simulink model "IEEE13NF_bal"  (Simulink 8.5)
settings: Solver=ode4  StartTime=0.0  StopTime=8  FixedStep=Ts  RelTol=1e-3
PreLoadFcn:
  | Ts=0.01;
PostLoadFcn:
  | Ts=0.01;
InitFcn:
  | Ts=0.01;
StartFcn:
  | Ts=0.01;
libraries: dspindex x5, opal_lib x2, rtlab x2, rtlab_phasor x1
settings Model: Creator=ZhiqiZhao  LastModifiedBy=Jaimie.Swartz
settings DebuggingCC: SolverPrmCheckMsg=warning  FcnCallInpInsideContextMsg=EnableAllAsWarning

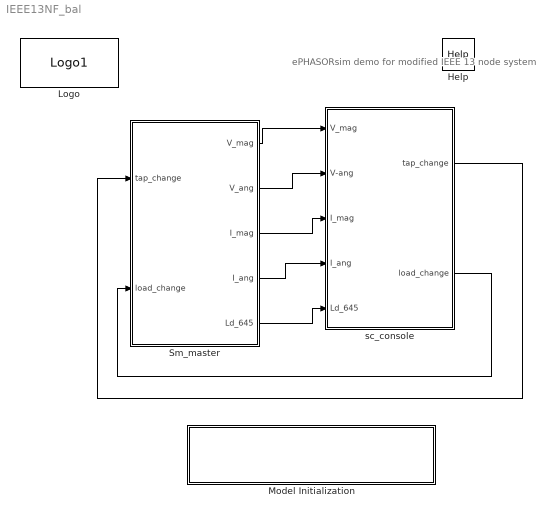
== system IEEE13NF_bal ==
  note: ePHASORsim demo for
      | modified IEEE 13 node system
  Help : opal_lib/Help  docfile=../help/ePH_IEEE13.html
  Logo : opal_lib/Logo1  vide=[]
  Model Initialization : Subsystem  mask(Model Functions){InitFcnX=Ts=0.01;, prel=on, posl=on, inif=on, strf=on}
      mask prompts: InitFcnX "Initialisation"; prel "Preload Function"; posl "PostLoad Function"; inif "InitFcn"; strf "StartFcn"
      mask init:
      | currentBlock = gcb;
      | root = bdroot(currentBlock);
      | 
      | if ~strcmp(get_param(root,'BlockDiagramType'),'library')
      |     if prel==1
      |         set_param(root, 'PreLoadFcn', InitFcnX);
      |     else
      |         set_param(root, 'PreLoadFcn', '');
      |     end
      |     if inif==1
      |         set_param(root, 'InitFcn', InitFcnX);
      |     else
      |         set_param(root, 'InitFcn', '');
      |     end
      |     if strf==1
      |         set_param(root, 'StartFcn', InitFcnX);
      |     else
      |         set_param(root, 'StartFcn', '');
      |     end
      |     if posl==1
      |         set_param(root, 'PostLoadFcn', InitFcnX);
      |     else
      |         set_param(root, 'PostLoadFcn', '');
      |     end
      | end
      | 
      | pos = get_param(currentBlock, 'Position');
      | width = pos(3) - pos(1); height = pos(4) - pos(2);
      | txt = [ upper(root) '\n' '- InitFcn. . . . . '  get_param(root, 'InitFcn') ];
      settings: CopyFcn=set_param(gcb,'LinkStatus','none')
      mask Display: text(5, height*0.5, txt, 'horizontalAlignment', 'left', 'verticalAlignment', 'middle') ;
  Sm_master : Subsystem
  sc_console : Subsystem
  wires:
  sc_console/1(tap_change) -> Sm_master/1(tap_change)
  sc_console/2(load_change) -> Sm_master/2(load_change)
  Sm_master/1(V_mag) -> sc_console/1(V_mag)
  Sm_master/2(V_ang) -> sc_console/2(V-ang)
  Sm_master/3(I_mag) -> sc_console/3(I_mag)
  Sm_master/4(I_ang) -> sc_console/4(I_ang)
  Sm_master/5(Ld_645) -> sc_console/5(Ld_645)

== system IEEE13NF_bal/Model Initialization ==

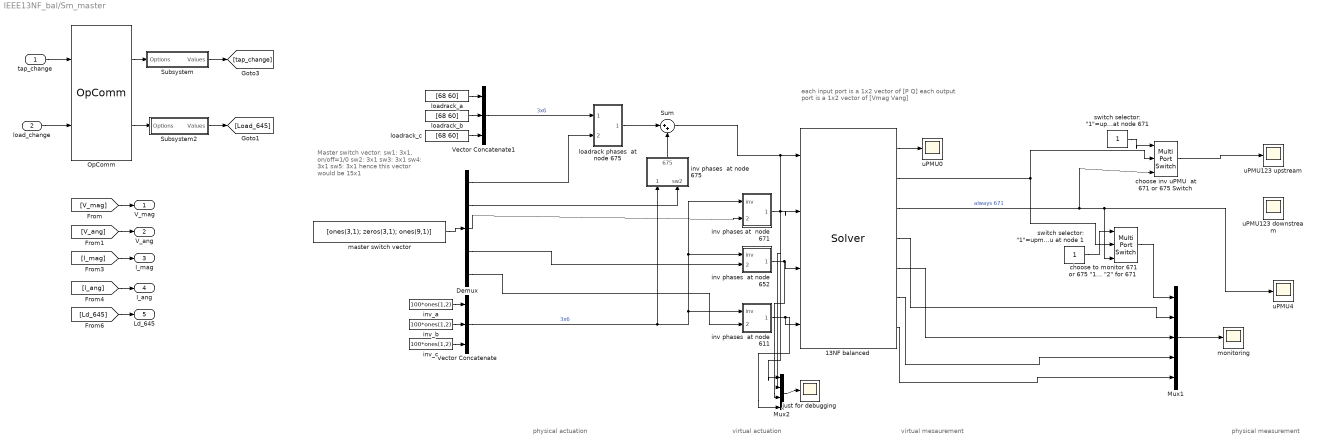
== system IEEE13NF_bal/Sm_master ==
  note: Master switch vector:
      | sw1: 3x1, on/off=1/0
      | sw2: 3x1
      | sw3: 3x1
      | sw4: 3x1
      | sw5: 3x1
      | hence this vector would be 15x1
  note: virtual actuation
  note: virtual mesaurement
  note: physical measurement
  note: physical actuation
  note: each input port is a 1x2 vector of [P Q]
      | each output port is a 1x2 vector of [Vmag Vang]
  tap_change : Inport
  load_change : Inport  Port=2
  13NF balanced : rtlab_phasor/Solver  epname=System  extension=Excel  xls='016_GB_IEEE13_balance_all_ver2_OPAL.xls'  raw='4992b.raw'  dyr='4992b.dyr'  cyme='ieee13.sxst'  powerfactory='network.dgs'  builtin=on  cyme_pf=''  cyme_unbalanced=on  lazy_netlist=on  capidir='CAPI'  fmudir='FMU'  capiprefix=capicomp_  fmuprefix=fmucomp_  logging=off  sim_mode=Dynamic simulation only (without power-flow)  pf_max_it=100  pf_tol_v=0.00000001  pf_flat_start=off  pf_smart_start=off  pf_export=on  np=1  exporty=off  dt=Ts  optim_threads=off  perflog_on=off  script_activate_postinit=on  script_postinit_name='manual_python_integration_13NFbal.py'
  Demux : Demux  Outputs=5
  Mux1 : Mux  Inputs=5
  Mux2 : Mux
  OpComm : rtlab/OpComm  nbport=2  groupe_acq=1  subsys_rate=0  st=0  Synchronization=on  Interpolation=on  Threshold=1.0  Missed_Data=off  Sim_Time=off  Samples=off  dynSigOut=off  from_console=1  warning_done=off  writeOpCommFile=off  Offset=off
  Subsystem : Subsystem
  Subsystem2 : Subsystem
  Sum : Sum  Inputs=|++
  Vector Concatenate : Concatenate  NumInputs=3  Mode=Multidimensional array  ConcatenateDimension=2
  Vector Concatenate1 : Concatenate  NumInputs=3  Mode=Multidimensional array  ConcatenateDimension=2
  choose inv uPMU  at 671 or 675 Switch : MultiPortSwitch  Inputs=2
  "choose to monitor 671 or 675 \"1\" for 675 \"2\" for 671" : MultiPortSwitch  Inputs=2
  inv phases  at node 675 : Subsystem
  inv phases  at node 611 : Subsystem
  inv phases  at node 652 : Subsystem
  inv phases at  node 671 : Subsystem
  inv_a : Constant  Value=100*ones(1,2)
  inv_b : Constant  Value=100*ones(1,2)
  inv_c : Constant  Value=100*ones(1,2)
  just for debugging : Scope
      settings: SaveName=ScopeData22
  loadrack phases  at node 675 : Subsystem
  loadrack_a : Constant  Value=[68 60]
  loadrack_b : Constant  Value=[68 60]
  loadrack_c : Constant  Value=[68 60]
  master switch vector : Constant  Value=[ones(3,1); zeros(3,1); ones(9,1)]
  monitoring : Scope
      settings: SaveName=ScopeData21
  "switch selector: \"1\"=upmu at node 675 \"2\"=upmu at node 1" : Constant
  "switch selector: \"1\"=upmu at node 675 \"2\"=upmu at node 671" : Constant
  uPMU0 : Scope
  uPMU123 downstream : Scope
      settings: SaveName=ScopeData2
  uPMU123 upstream : Scope
      settings: SaveName=ScopeData17
  uPMU4 : Scope
      settings: SaveName=ScopeData16
  V_mag : Outport
  V_ang : Outport  Port=2
  I_mag : Outport  Port=3
  I_ang : Outport  Port=4
  Ld_645 : Outport  Port=5
  wires:
  tap_change/1 -> OpComm/1
  load_change/1 -> OpComm/2
  OpComm/1 -> Subsystem/1(Options)
  OpComm/2 -> Subsystem2/1(Options)
  Subsystem/1(Values) -> [tap_change]
  Subsystem2/1(Values) -> [Load_645]
  [Ld_645] -> Ld_645/1
  [I_ang] -> I_ang/1
  [I_mag] -> I_mag/1
  [V_ang] -> V_ang/1
  [V_mag] -> V_mag/1
  loadrack_a/1 -> Vector Concatenate1/1
  loadrack_b/1 -> Vector Concatenate1/2
  loadrack_c/1 -> Vector Concatenate1/3
  Vector Concatenate1/1 -> loadrack phases  at node 675/1(loadrack)  "3x6"
  inv_a/1 -> Vector Concatenate/1
  inv_b/1 -> Vector Concatenate/2
  inv_c/1 -> Vector Concatenate/3
  Sum/1 -> Mux2/1, 13NF balanced/1
  Vector Concatenate/1 -> inv phases  at node 675/1(loadrack), inv phases  at node 611/1(inv), inv phases at  node 671/1(inv), inv phases  at node 652/1(inv)  "3x6"
  inv phases at  node 671/1(671) -> Mux2/2, 13NF balanced/2
  inv phases  at node 652/1(652) -> Mux2/3, 13NF balanced/3
  inv phases  at node 611/1(611) -> Mux2/4, 13NF balanced/4
  13NF balanced/7 -> Mux1/5
  13NF balanced/5 -> Mux1/3
  13NF balanced/4 -> Mux1/2
  "switch selector: \"1\"=upmu at node 675 \"2\"=upmu at node 671"/1 -> choose inv uPMU  at 671 or 675 Switch/1
  13NF balanced/1 -> uPMU0/1
  choose inv uPMU  at 671 or 675 Switch/1 -> uPMU123 upstream/1
  13NF balanced/3 -> choose inv uPMU  at 671 or 675 Switch/3, "choose to monitor 671 or 675 \"1\" for 675 \"2\" for 671"/3, uPMU4/1  "always 671"
  "choose to monitor 671 or 675 \"1\" for 675 \"2\" for 671"/1 -> Mux1/1
  13NF balanced/6 -> Mux1/4
  Mux1/1 -> monitoring/1
  ? -> uPMU123 downstream/1
  loadrack phases  at node 675/1(675) -> Sum/1
  inv phases  at node 675/1(675) -> Sum/2
  master switch vector/1 -> Demux/1
  Demux/1 -> loadrack phases  at node 675/2(sw1)
  Demux/2 -> inv phases  at node 675/2(sw2)
  Demux/3 -> inv phases at  node 671/2(sw3)
  Demux/4 -> inv phases  at node 652/2(sw4)
  Demux/5 -> inv phases  at node 611/2(sw5)
  Mux2/1 -> just for debugging/1
  "switch selector: \"1\"=upmu at node 675 \"2\"=upmu at node 1"/1 -> "choose to monitor 671 or 675 \"1\" for 675 \"2\" for 671"/1
  13NF balanced/2 -> "choose to monitor 671 or 675 \"1\" for 675 \"2\" for 671"/2, choose inv uPMU  at 671 or 675 Switch/2

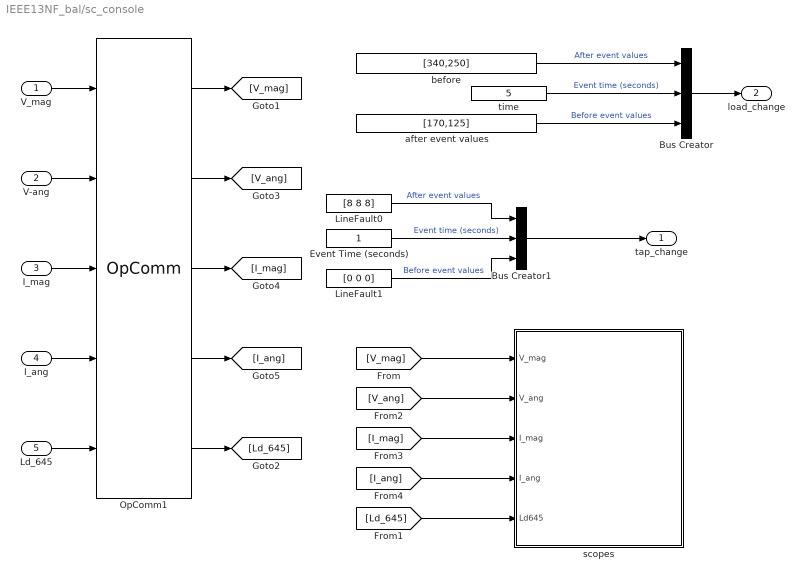
== system IEEE13NF_bal/sc_console ==
  V_mag : Inport
  V-ang : Inport  Port=2
  I_mag : Inport  Port=3
  I_ang : Inport  Port=4
  Ld_645 : Inport  Port=5
  Bus Creator : BusCreator  Inputs=3
  Bus Creator1 : BusCreator  Inputs=3
  Event Time (seconds) : Constant
  LineFault0 : Constant  Value=[8 8 8]
  LineFault1 : Constant  Value=[0 0 0]
  OpComm1 : rtlab/OpComm  nbport=5  groupe_acq=1  subsys_rate=0  st=0  Synchronization=on  Interpolation=on  Threshold=1.0  Missed_Data=off  Sim_Time=off  Samples=off  dynSigOut=off  from_console=0  warning_done=off  writeOpCommFile=off  Offset=off
  after event values : Constant  Value=[170,125]
  before : Constant  Value=[340,250]
  scopes : Subsystem
  time : Constant  Value=5
  tap_change : Outport
  load_change : Outport  Port=2
  wires:
  V-ang/1 -> OpComm1/2
  V_mag/1 -> OpComm1/1
  OpComm1/1 -> [V_mag]
  OpComm1/2 -> [V_ang]
  time/1 -> Bus Creator/2  "Event time (seconds)"
  Bus Creator/1 -> load_change/1
  LineFault0/1 -> Bus Creator1/1  "After event values"
  LineFault1/1 -> Bus Creator1/3  "Before event values"
  Event Time (seconds)/1 -> Bus Creator1/2  "Event time (seconds)"
  Bus Creator1/1 -> tap_change/1
  before/1 -> Bus Creator/1  "After event values"
  after event values/1 -> Bus Creator/3  "Before event values"
  OpComm1/5 -> [Ld_645]
  Ld_645/1 -> OpComm1/5
  I_mag/1 -> OpComm1/3
  I_ang/1 -> OpComm1/4
  OpComm1/4 -> [I_ang]
  OpComm1/3 -> [I_mag]
  [V_mag] -> scopes/1(V_mag)
  [V_ang] -> scopes/2(V_ang)
  [I_mag] -> scopes/3(I_mag)
  [I_ang] -> scopes/4(I_ang)
  [Ld_645] -> scopes/5(Ld645)

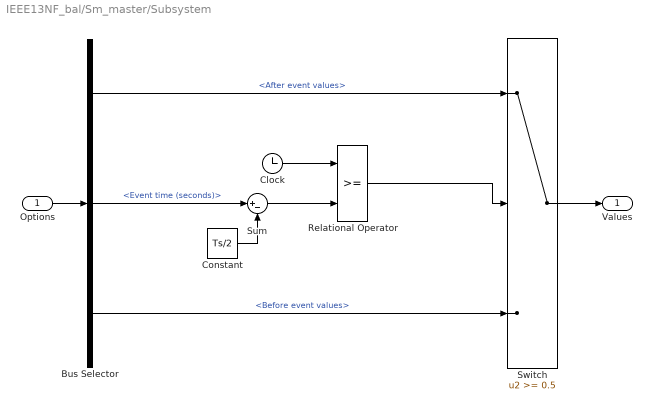
== system IEEE13NF_bal/Sm_master/Subsystem ==
  Options : Inport
  Bus Selector : BusSelector  OutputSignals=After event values,Event time (seconds),Before event values
  Clock : Clock
  Constant : Constant  Value=Ts/2
  Relational Operator : RelationalOperator  OutDataTypeStr=boolean
  Sum : Sum  Inputs=|+-
  Switch : Switch  Threshold=0.5
  Values : Outport
  wires:
  Clock/1 -> Relational Operator/1
  Constant/1 -> Sum/2
  Sum/1 -> Relational Operator/2
  Bus Selector/2 -> Sum/1  "<Event time (seconds)>"
  Relational Operator/1 -> Switch/2
  Bus Selector/3 -> Switch/3  "<Before event values>"
  Bus Selector/1 -> Switch/1  "<After event values>"
  Switch/1 -> Values/1
  Options/1 -> Bus Selector/1

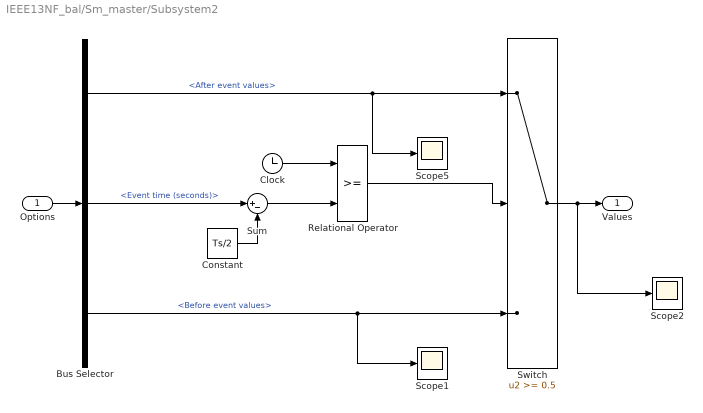
== system IEEE13NF_bal/Sm_master/Subsystem2 ==
  Options : Inport
  Bus Selector : BusSelector  OutputSignals=After event values,Event time (seconds),Before event values
  Clock : Clock
  Constant : Constant  Value=Ts/2
  Relational Operator : RelationalOperator  OutDataTypeStr=boolean
  Scope1 : Scope
      settings: SaveName=ScopeData14
  Scope2 : Scope
      settings: SaveName=ScopeData15
  Scope5 : Scope
      settings: SaveName=ScopeData13
  Sum : Sum  Inputs=|+-
  Switch : Switch  Threshold=0.5
  Values : Outport
  wires:
  Clock/1 -> Relational Operator/1
  Constant/1 -> Sum/2
  Sum/1 -> Relational Operator/2
  Bus Selector/2 -> Sum/1  "<Event time (seconds)>"
  Relational Operator/1 -> Switch/2
  Bus Selector/3 -> Switch/3, Scope1/1  "<Before event values>"
  Bus Selector/1 -> Switch/1, Scope5/1  "<After event values>"
  Switch/1 -> Values/1, Scope2/1
  Options/1 -> Bus Selector/1

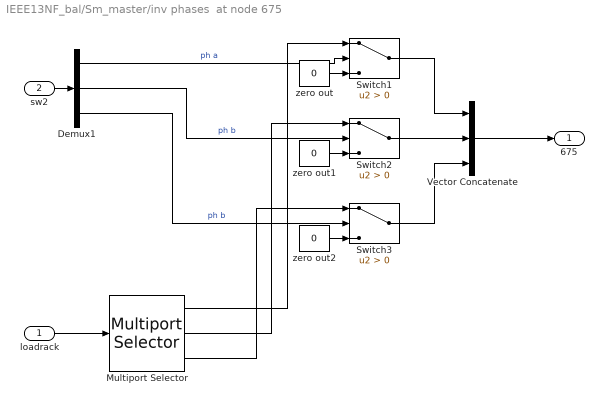
== system IEEE13NF_bal/Sm_master/inv phases  at node 675 ==
  loadrack : Inport
  sw2 : Inport  Port=2
  Demux1 : Demux  Outputs=3
  Multiport Selector : dspindex/Multiport Selector  rowsOrCols=Columns  idxCellArray={ 1, 2, 3 }  idxErrMode=Clip Index
  Switch1 : Switch  Criteria=u2 > Threshold
  Switch2 : Switch  Criteria=u2 > Threshold
  Switch3 : Switch  Criteria=u2 > Threshold
  Vector Concatenate : Concatenate  NumInputs=3  ConcatenateDimension=2
  zero out : Constant  Value=0
  zero out1 : Constant  Value=0
  zero out2 : Constant  Value=0
  675 : Outport
  wires:
  Demux1/3 -> Switch3/2  "ph b"
  zero out2/1 -> Switch3/3
  Demux1/1 -> Switch1/2  "ph a"
  zero out/1 -> Switch1/3
  loadrack/1 -> Multiport Selector/1
  Switch2/1 -> Vector Concatenate/2
  Switch1/1 -> Vector Concatenate/1
  Switch3/1 -> Vector Concatenate/3
  Vector Concatenate/1 -> 675/1
  Multiport Selector/2 -> Switch2/1
  Multiport Selector/1 -> Switch1/1
  Multiport Selector/3 -> Switch3/1
  Demux1/2 -> Switch2/2  "ph b"
  zero out1/1 -> Switch2/3
  sw2/1 -> Demux1/1

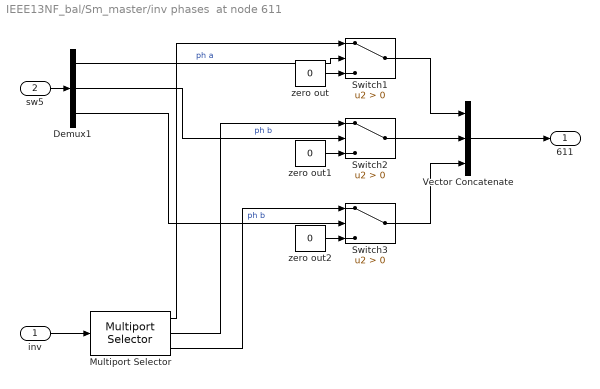
== system IEEE13NF_bal/Sm_master/inv phases  at node 611 ==
  inv : Inport
  sw5 : Inport  Port=2
  Demux1 : Demux  Outputs=3
  Multiport Selector : dspindex/Multiport Selector  rowsOrCols=Columns  idxCellArray={ 1, 2, 3 }  idxErrMode=Clip Index
  Switch1 : Switch  Criteria=u2 > Threshold
  Switch2 : Switch  Criteria=u2 > Threshold
  Switch3 : Switch  Criteria=u2 > Threshold
  Vector Concatenate : Concatenate  NumInputs=3  ConcatenateDimension=2
  zero out : Constant  Value=0
  zero out1 : Constant  Value=0
  zero out2 : Constant  Value=0
  611 : Outport
  wires:
  Demux1/3 -> Switch3/2  "ph b"
  zero out2/1 -> Switch3/3
  Demux1/1 -> Switch1/2  "ph a"
  zero out/1 -> Switch1/3
  Switch2/1 -> Vector Concatenate/2
  Switch1/1 -> Vector Concatenate/1
  Switch3/1 -> Vector Concatenate/3
  Vector Concatenate/1 -> 611/1
  Multiport Selector/2 -> Switch2/1
  Multiport Selector/1 -> Switch1/1
  Multiport Selector/3 -> Switch3/1
  Demux1/2 -> Switch2/2  "ph b"
  zero out1/1 -> Switch2/3
  sw5/1 -> Demux1/1
  inv/1 -> Multiport Selector/1

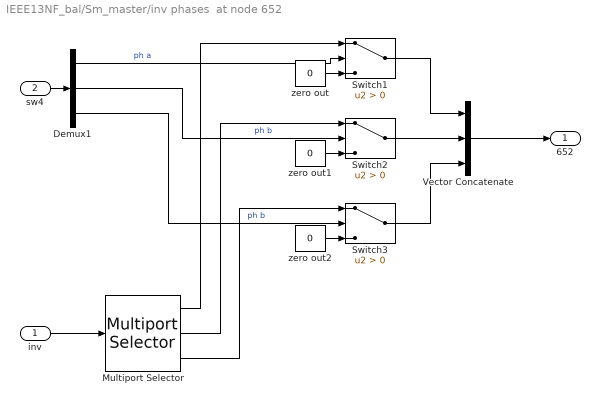
== system IEEE13NF_bal/Sm_master/inv phases  at node 652 ==
  inv : Inport
  sw4 : Inport  Port=2
  Demux1 : Demux  Outputs=3
  Multiport Selector : dspindex/Multiport Selector  rowsOrCols=Columns  idxCellArray={ 1, 2, 3 }  idxErrMode=Clip Index
  Switch1 : Switch  Criteria=u2 > Threshold
  Switch2 : Switch  Criteria=u2 > Threshold
  Switch3 : Switch  Criteria=u2 > Threshold
  Vector Concatenate : Concatenate  NumInputs=3  ConcatenateDimension=2
  zero out : Constant  Value=0
  zero out1 : Constant  Value=0
  zero out2 : Constant  Value=0
  652 : Outport
  wires:
  Demux1/3 -> Switch3/2  "ph b"
  zero out2/1 -> Switch3/3
  Demux1/1 -> Switch1/2  "ph a"
  zero out/1 -> Switch1/3
  inv/1 -> Multiport Selector/1
  Switch2/1 -> Vector Concatenate/2
  Switch1/1 -> Vector Concatenate/1
  Switch3/1 -> Vector Concatenate/3
  Vector Concatenate/1 -> 652/1
  Multiport Selector/2 -> Switch2/1
  Multiport Selector/1 -> Switch1/1
  Multiport Selector/3 -> Switch3/1
  Demux1/2 -> Switch2/2  "ph b"
  zero out1/1 -> Switch2/3
  sw4/1 -> Demux1/1

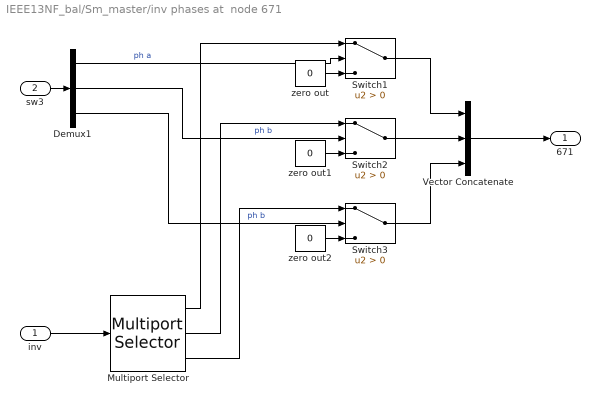
== system IEEE13NF_bal/Sm_master/inv phases at  node 671 ==
  inv : Inport
  sw3 : Inport  Port=2
  Demux1 : Demux  Outputs=3
  Multiport Selector : dspindex/Multiport Selector  rowsOrCols=Columns  idxCellArray={ 1, 2, 3 }  idxErrMode=Clip Index
  Switch1 : Switch  Criteria=u2 > Threshold
  Switch2 : Switch  Criteria=u2 > Threshold
  Switch3 : Switch  Criteria=u2 > Threshold
  Vector Concatenate : Concatenate  NumInputs=3  ConcatenateDimension=2
  zero out : Constant  Value=0
  zero out1 : Constant  Value=0
  zero out2 : Constant  Value=0
  671 : Outport
  wires:
  Demux1/3 -> Switch3/2  "ph b"
  zero out2/1 -> Switch3/3
  Demux1/1 -> Switch1/2  "ph a"
  zero out/1 -> Switch1/3
  inv/1 -> Multiport Selector/1
  Switch2/1 -> Vector Concatenate/2
  Switch1/1 -> Vector Concatenate/1
  Switch3/1 -> Vector Concatenate/3
  Vector Concatenate/1 -> 671/1
  Multiport Selector/2 -> Switch2/1
  Multiport Selector/1 -> Switch1/1
  Multiport Selector/3 -> Switch3/1
  Demux1/2 -> Switch2/2  "ph b"
  zero out1/1 -> Switch2/3
  sw3/1 -> Demux1/1

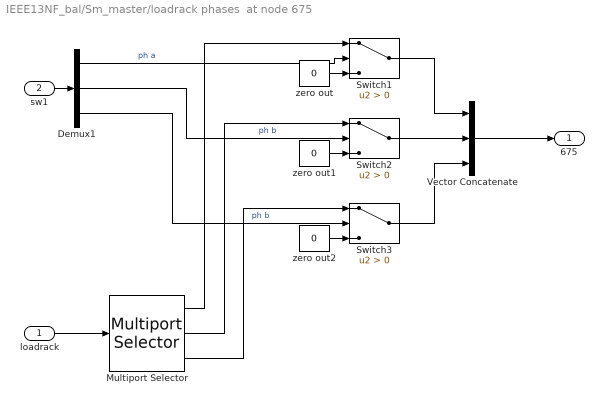
== system IEEE13NF_bal/Sm_master/loadrack phases  at node 675 ==
  loadrack : Inport
  sw1 : Inport  Port=2
  Demux1 : Demux  Outputs=3
  Multiport Selector : dspindex/Multiport Selector  rowsOrCols=Columns  idxCellArray={ 1, 2, 3 }  idxErrMode=Clip Index
  Switch1 : Switch  Criteria=u2 > Threshold
  Switch2 : Switch  Criteria=u2 > Threshold
  Switch3 : Switch  Criteria=u2 > Threshold
  Vector Concatenate : Concatenate  NumInputs=3  ConcatenateDimension=2
  zero out : Constant  Value=0
  zero out1 : Constant  Value=0
  zero out2 : Constant  Value=0
  675 : Outport
  wires:
  Demux1/3 -> Switch3/2  "ph b"
  zero out2/1 -> Switch3/3
  Demux1/1 -> Switch1/2  "ph a"
  zero out/1 -> Switch1/3
  loadrack/1 -> Multiport Selector/1
  Switch2/1 -> Vector Concatenate/2
  Switch1/1 -> Vector Concatenate/1
  Switch3/1 -> Vector Concatenate/3
  Vector Concatenate/1 -> 675/1
  Multiport Selector/2 -> Switch2/1
  Multiport Selector/1 -> Switch1/1
  Multiport Selector/3 -> Switch3/1
  Demux1/2 -> Switch2/2  "ph b"
  zero out1/1 -> Switch2/3
  sw1/1 -> Demux1/1

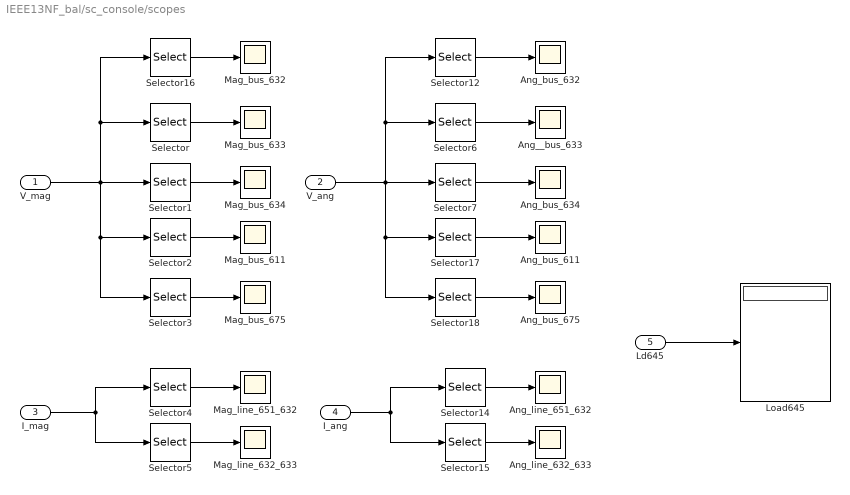
== system IEEE13NF_bal/sc_console/scopes ==
  V_mag : Inport
  V_ang : Inport  Port=2
  I_mag : Inport  Port=3
  I_ang : Inport  Port=4
  Ld645 : Inport  Port=5
  Ang__bus_633 : Scope
      settings: YMin=0.92  YMax=1.07  SaveName=ScopeData8
  Ang_bus_{611,632,634,675} (4 alike) : Scope
      Ang_bus_611 settings: YMin=0.92  YMax=1.07  SaveName=ScopeData10
      Ang_bus_632 settings: YMin=0.92  YMax=1.07  SaveName=ScopeData18
      Ang_bus_634 settings: YMin=0.92  YMax=1.07  SaveName=ScopeData9
      Ang_bus_675 settings: YMin=0.92  YMax=1.07  SaveName=ScopeData11
  Ang_line_632_633 : Scope
      settings: YMin=0.92  YMax=1.07  SaveName=ScopeData20
  Ang_line_651_632 : Scope
      settings: YMin=0.92  YMax=1.07
  Load645 : Display
  Mag_bus_{611,632..634,675} (5 alike) : Scope
      Mag_bus_611 settings: YMin=0.92  YMax=1.07  SaveName=ScopeData6
      Mag_bus_632 settings: YMin=0.92  YMax=1.07  SaveName=ScopeData3
      Mag_bus_633 settings: YMin=0.92  YMax=1.07  SaveName=ScopeData4
      Mag_bus_634 settings: YMin=0.92  YMax=1.07  SaveName=ScopeData5
      Mag_bus_675 settings: YMin=0.92  YMax=1.07  SaveName=ScopeData7
  Mag_line_632_633 : Scope
      settings: YMin=0.92  YMax=1.07  SaveName=ScopeData19
  Mag_line_651_632 : Scope
      settings: YMin=0.92  YMax=1.07  SaveName=ScopeData12
  Selector : Selector  InputPortWidth=13  Indices=[1 2 3]
  Selector1 : Selector  InputPortWidth=13  Indices=[4 5 6]
  Selector12 : Selector  InputPortWidth=13  Indices=[11 12 13]
  Selector14 : Selector  InputPortWidth=6  Indices=[1 2 3]
  Selector15 : Selector  InputPortWidth=6  Indices=[4 5 6]
  Selector16 : Selector  InputPortWidth=13  Indices=[11 12 13]
  Selector17 : Selector  InputPortWidth=13  Indices=[7]
  Selector18 : Selector  InputPortWidth=13  Indices=[8 9 10]
  Selector2 : Selector  InputPortWidth=13  Indices=[7]
  Selector3 : Selector  InputPortWidth=13  Indices=[8 9 10]
  Selector4 : Selector  InputPortWidth=6  Indices=[1 2 3]
  Selector5 : Selector  InputPortWidth=6  Indices=[4 5 6]
  Selector6 : Selector  InputPortWidth=13  Indices=[1 2 3]
  Selector7 : Selector  InputPortWidth=13  Indices=[4 5 6]
  wires:
  Selector/1 -> Mag_bus_633/1
  Selector1/1 -> Mag_bus_634/1
  Selector2/1 -> Mag_bus_611/1
  Selector3/1 -> Mag_bus_675/1
  V_mag/1 -> Selector1/1, Selector3/1, Selector2/1, Selector/1, Selector16/1
  Ld645/1 -> Load645/1
  Selector4/1 -> Mag_line_651_632/1
  Selector14/1 -> Ang_line_651_632/1
  I_ang/1 -> Selector14/1, Selector15/1
  Selector16/1 -> Mag_bus_632/1
  I_mag/1 -> Selector5/1, Selector4/1
  Selector5/1 -> Mag_line_632_633/1
  Selector15/1 -> Ang_line_632_633/1
  V_ang/1 -> Selector12/1, Selector6/1, Selector17/1, Selector18/1, Selector7/1
  Selector12/1 -> Ang_bus_632/1
  Selector6/1 -> Ang__bus_633/1
  Selector7/1 -> Ang_bus_634/1
  Selector17/1 -> Ang_bus_611/1
  Selector18/1 -> Ang_bus_675/1
